simulink model "lab1_hw_closedloop"  (R2018b)
settings: Solver=ode1  StartTime=0.0  StopTime=5  FixedStep=0.002  RelTol=1e-3  EnableMultiTasking=on
undefined symbols (not defined in the file or in its folder): HIL
libraries: quarc_library x4
settings Model: SimulationMode=external  ExtModeTrigDuration=50001  Creator=Mounir  LastModifiedBy=edod2243
settings SolverCC: PositivePriorityOrder=on
settings DataIOCC: LimitDataPoints=on  SaveFormat=Array  SaveOutput=off  SaveTime=off
settings OptimizationCC: LifeSpan=inf
settings DebuggingCC: SolverPrmCheckMsg=warning  AllowSymbolicDim=off  SFUnexpectedBacktrackingDiag=warning  SFNoUnconditionalDefaultTransitionDiag=warning  SFExecutionAtInitializationDiag=none
settings HardwareCC: ProdBitPerPointer=32  ProdBitPerSizeT=32  ProdBitPerPtrDiffT=32  ProdLargestAtomicFloat=None  ProdIntDivRoundTo=Undefined  ProdEndianess=Unspecified  ProdWordSize=32  ProdHWDeviceType=32-bit Generic
settings ModelReferenceCC: PropagateSignalLabelsOutOfModel=off
settings SFSimCC: SimUseLocalCustomCode=off
settings RTWCC: SystemTargetFile=quarc_win64.tlc  TemplateMakefile=quarc_default_tmf  Description=QUARC Win64 Target  RTWUseLocalCustomCode=off
settings CodeAppCC: StateflowObjectComments=on
settings STFCustomTargetCC: TargetPreCompLibLocation=C:\PROGRA~3\QUARC\lib\2018b\win64\release  ConcurrentExecutionCompliant=on  GeneratePreprocessorConditionals=Disable all  CombineOutputUpdateFcns=on  SystemTargetFile=quarc_win64.tlc
settings GRTTargetCC: TargetPreCompLibLocation=C:\PROGRA~3\QUARC\lib\2018b\win64\release  TargetLangStandard=C89/C90 (ANSI)  ParMdlRefBuildCompliant=off  CompOptLevelCompliant=off  GeneratePreprocessorConditionals=Disable all  MatFileLogging=off  CPPClassGenCompliant=off  UseToolchainInfoCompliant=off  ExtMode=on  ExtModeMexFile=quarc_comm
settings ConfigComp: CovMetricSettings=dw  CovHtmlReporting=on  CovSaveCumulativeToWorkspaceVar=on  CovSaveSingleToWorkspaceVar=on  CovExternalEMLEnable=off  CovSFcnEnable=off

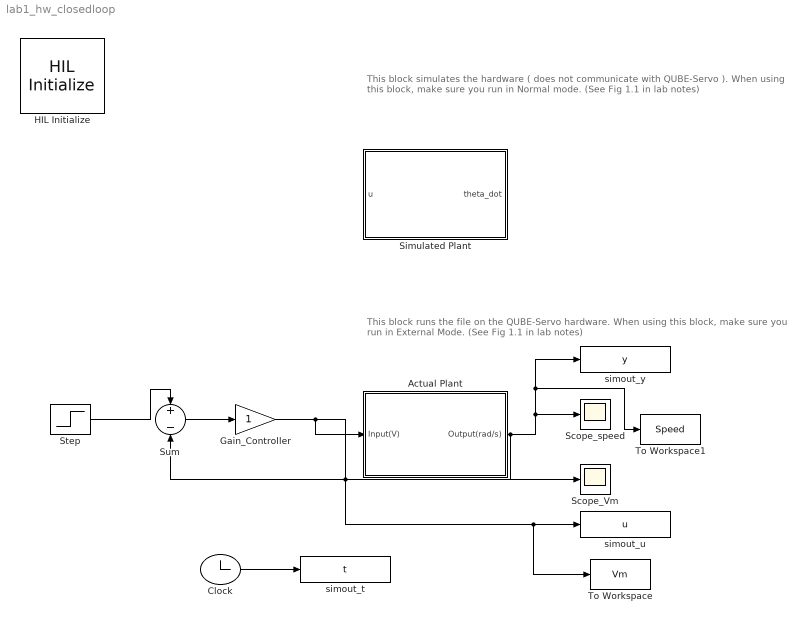
== system lab1_hw_closedloop ==
  note: This block simulates the hardware ( does not communicate with QUBE-Servo ).
      | When using this block, make sure you run in Normal mode. (See Fig 1.1 in lab notes)
  note: This block runs the file on the QUBE-Servo hardware.
      | When using this block, make sure you run in External Mode. (See Fig 1.1 in lab notes)
  Actual Plant : Subsystem
  Clock : Clock
  Gain_Controller : Gain
  HIL Initialize : quarc_library/Data Acquisition/Generic/Configuration/HIL Initialize  Priority=-99  object_name=HIL-1  board_type=qube_servo_usb  board_number=0  board_options=d0=pwm;d1=pwm;led=auto;update_rate=normal;decimation=1  exclusive=off  active=off  hardware_clocks=[0]  clock_modes=[]  initial_clock_frequencies=[]  set_clock_params_at_start=off  set_clock_params_at_switch_in=off  set_clock_frequencies_at_start=off  set_clock_frequencies_at_switch_in=off  analog_input_channels=[]  analog_input_configurations=[]  analog_input_maximums=[]  analog_input_minimums=[]  set_analog_input_params_at_start=off  set_analog_input_params_at_switch_in=off  analog_output_channels=[0:1]  analog_output_maximums=10  analog_output_minimums=-10  initial_analog_outputs=[0]  final_analog_outputs=[0]  watchdog_analog_outputs=0  set_analog_output_params_at_start=on  set_analog_output_params_at_switch_in=off  set_analog_outputs_at_start=on  set_analog_outputs_at_switch_in=off  set_analog_outputs_at_terminate=on  set_analog_outputs_at_switch_out=off  set_analog_outputs_on_watchdog=off  digital_input_channels=[]  digital_output_channels=[]  digital_output_configuration=[]  initial_digital_outputs=[]  final_digital_outputs=[]  watchdog_digital_outputs=[]  set_digital_output_params_at_start=off  set_digital_output_params_at_switch_in=off  set_digital_outputs_at_start=off  set_digital_outputs_at_switch_in=off  set_digital_outputs_at_terminate=off  set_digital_outputs_at_switch_out=off  set_digital_outputs_on_watchdog=off  encoder_channels=[0:1]  quadrature=[4]  encoder_filter_frequency=[]  initial_encoder_counts=[0]  set_encoder_params_at_start=on  set_encoder_params_at_switch_in=off  set_encoder_counts_at_start=on  set_encoder_counts_at_switch_in=off  pwm_channels=[]  pwm_modes=[]  pwm_frequency=[]  pwm_configuration=[]  pwm_alignment=[]  pwm_polarity=[]  pwm_leading_deadband=[]  pwm_trailing_deadband=[]  initial_pwm_outputs=[]  final_pwm_outputs=[]  watchdog_pwm_outputs=[]  set_pwm_params_at_start=off  set_pwm_params_at_switch_in=off  set_pwm_outputs_at_start=off  set_pwm_outputs_at_switch_in=off  set_pwm_outputs_at_terminate=off  set_pwm_outputs_at_switch_out=off  set_pwm_outputs_on_watchdog=off  other_output_channels=[]  initial_other_outputs=[]  final_other_outputs=[]  watchdog_other_outputs=[]  set_other_outputs_at_start=off  set_other_outputs_at_switch_in=off  set_other_outputs_at_terminate=off  set_other_outputs_at_switch_out=off  set_other_outputs_on_watchdog=off
  Scope_Vm : Scope
  Scope_speed : Scope
  Simulated Plant : Subsystem
      mask Display:
      | %image('Qube.jpg')
      | port_label('input', 1, 'Input(V)')
      | port_label('output', 1, 'Output(rad/s)')
  Step : Step  After=10  SampleTime=0
  Sum : Sum  Inputs=+-
  To Workspace : ToWorkspace  VariableName=Vm  SampleTime=-1
  To Workspace1 : ToWorkspace  VariableName=Speed  SampleTime=-1
  simout_t : ToWorkspace  VariableName=t  SampleTime=-1
  simout_u : ToWorkspace  VariableName=u  SampleTime=-1
  simout_y : ToWorkspace  VariableName=y  SampleTime=-1
  wires:
  Step/1 -> Sum/1
  Sum/1 -> Gain_Controller/1
  Gain_Controller/1 -> Scope_Vm/1, To Workspace/1, simout_u/1, Actual Plant/1(Input(V))
  Actual Plant/1(Output(rad/s)) -> Scope_speed/1, To Workspace1/1, simout_y/1, Sum/2
  Clock/1 -> simout_t/1

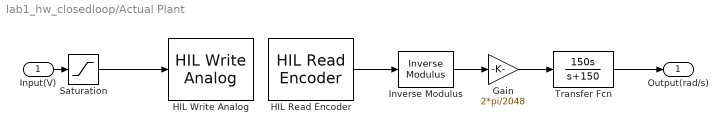
== system lab1_hw_closedloop/Actual Plant ==
  Input(V) : Inport
  Gain : Gain  Gain=2*pi/2048
  HIL Read Encoder : quarc_library/Data Acquisition/Generic/Immediate I//O/HIL Read Encoder  object_name=HIL-1  channels=0  sample_time=qc_get_step_size  active=on  vector_output=off  data_type_mode=Inherit via back propagation  data_type=double
  HIL Write Analog : quarc_library/Data Acquisition/Generic/Immediate I//O/HIL Write Analog  object_name=HIL-1  channels=0  sample_time=-1  active=off  vector_input=off
  Inverse Modulus : quarc_library/Discontinuities/Inverse Modulus  modulus=65535  output_derivative=off  output_revolutions=off  max_x=Inf  min_x=-Inf
  Saturation : Saturate  UpperLimit=10  LowerLimit=-10
  Transfer Fcn : TransferFcn  Numerator=[150 0]  Denominator=[1 150]
  Output(rad/s) : Outport
  wires:
  HIL Read Encoder/1 -> Inverse Modulus/1
  Input(V)/1 -> Saturation/1
  Inverse Modulus/1 -> Gain/1
  Gain/1 -> Transfer Fcn/1
  Transfer Fcn/1 -> Output(rad/s)/1
  Saturation/1 -> HIL Write Analog/1

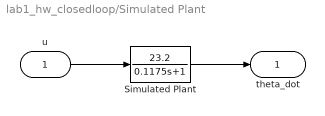
== system lab1_hw_closedloop/Simulated Plant ==
  u : Inport
  Simulated Plant : TransferFcn  Numerator=[23.2]  Denominator=[0.1175 1]
  theta_dot : Outport
  wires:
  Simulated Plant/1 -> theta_dot/1
  u/1 -> Simulated Plant/1
